simulink model "stateSpace"  (Simulink 8.6)
settings: Solver=ode45  StartTime=0  StopTime=9.424780e-04  MaxStep=1.000000e-07  RelTol=1e-3
undefined symbols (not defined in the file or in its folder): clarinet, flute, oboe
settings Model: Creator=Dan  LastModifiedBy=cobydavis
settings DataIOCC: LimitDataPoints=off  MaxDataPoints=500  LoadExternalInput=on  SaveFormat=StructureWithTime  ReturnWorkspaceOutputs=on
settings DebuggingCC: AlgebraicLoopMsg=none  SolverPrmCheckMsg=none  FcnCallInpInsideContextMsg=EnableAllAsWarning

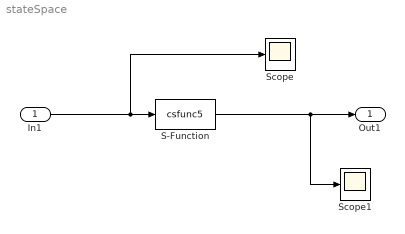
== system stateSpace ==
  In1 : Inport
  S-Function : S-Function  FunctionName=csfunc5  Parameters=flute,oboe,clarinet  SFunctionDeploymentMode=off  EnableBusSupport=off
  Scope : Scope
  Scope1 : Scope
  Out1 : Outport
  wires:
  S-Function/1 -> Scope1/1, Out1/1
  In1/1 -> Scope/1, S-Function/1
